simulink model "pasp_reordertest"  (Simulink 6.2)
settings: Solver=ode45  StartTime=0.0  StopTime=30000  RelTol=1e-3
undefined symbols (not defined in the file or in its folder): iBOB
libraries: xbsIndex_r3 x1464, casper_library x144, xps_library x60
(part 2 of 13)

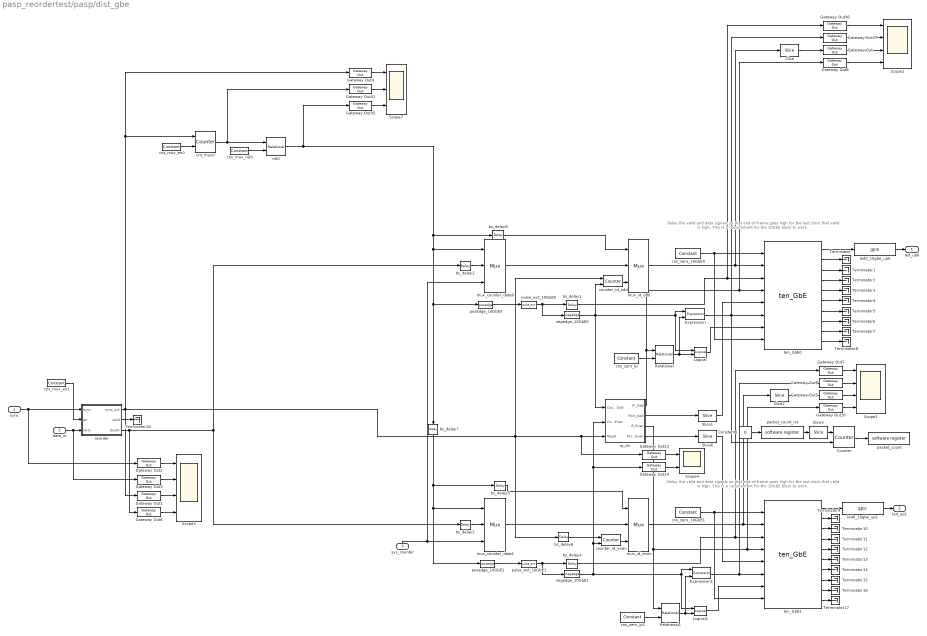
== system pasp_reordertest/pasp/dist_gbe ==
  note: Delay the valid and data signals so that
      | end-of-frame goes high for the last clock
      | that valid is high. This is a requirement for
      | the 10GbE block to work.
  note: Delay the valid and data signals so that
      | end-of-frame goes high for the last clock
      | that valid is high. This is a requirement for
      | the 10GbE block to work.
  sync : Inport  Port=1  LatchInput=off
  data_in : Inport  Port=2  LatchInput=off
  sys_counter : Inport  Orientation=up  Port=3  LatchInput=off
  Constant6 : Constant  Value=0
  Counter : xbsIndex_r3/Counter  cnt_type=Free Running  n_bits=32  bin_pt=0  arith_type=Unsigned  start_count=0  cnt_to=Inf  cnt_by_val=1  operation=Up  explicit_period=off  period=1  load_pin=off  rst=on  en=on  dbl_ovrd=off  show_param=off  use_rpm=on  gen_core=off
      settings: xl_area=[0, 0, 0, 0, 0, 0, 0]
  Expression : xbsIndex_r3/Expression  expression=a & ~b  precision=Full  arith_type=Unsigned  n_bits=8  bin_pt=2  align_bp=on  latency=0  explicit_period=off  period=1  en=off  dbl_ovrd=off  show_param=off
      settings: xl_area=[0, 0, 0, 0, 0, 0, 0]
  Expression1 : xbsIndex_r3/Expression  expression=a & ~b  precision=Full  arith_type=Unsigned  n_bits=8  bin_pt=2  align_bp=on  latency=0  explicit_period=off  period=1  en=off  dbl_ovrd=off  show_param=off
      settings: xl_area=[0, 0, 0, 0, 0, 0, 0]
  Gateway Out{,1..10,13..14,31,35..37} (17 alike) : xbsIndex_r3/Gateway Out  output_type=Double  nbits=8  bin_pt=6  arith_type=Boolean  quantization=Truncate  overflow=Wrap  hdl_port=on  timing_constraint=None  locs_specified=off  LOCs={}  needs_fixed_name=off  show_param=off
      settings: xl_area=[0, 0, 0, 0, 0, 0, 0]
  Logical : xbsIndex_r3/Logical  logical_function=AND  inputs=2  precision=Full  arith_type=Unsigned  n_bits=8  bin_pt=2  align_bp=on  latency=0  explicit_period=off  period=1  en=off  dbl_ovrd=off  show_param=off
      settings: xl_area=[0, 0, 0, 0, 0, 0, 0]
  Logical1 : xbsIndex_r3/Logical  logical_function=AND  inputs=2  precision=Full  arith_type=Unsigned  n_bits=8  bin_pt=2  align_bp=on  latency=0  explicit_period=off  period=1  en=off  dbl_ovrd=off  show_param=off
      settings: xl_area=[0, 0, 0, 0, 0, 0, 0]
  Relational : xbsIndex_r3/Relational  mode=a=b  latency=1  explicit_period=off  period=1  en=off  dbl_ovrd=off  show_param=off
      settings: xl_area=[0, 0, 0, 0, 0, 0, 0]
  Relational1 : xbsIndex_r3/Relational  mode=a=b  latency=1  explicit_period=off  period=1  en=off  dbl_ovrd=off  show_param=off
      settings: xl_area=[0, 0, 0, 0, 0, 0, 0]
  Scope1 : Scope  NumInputPorts=4
      settings: TimeRange=10000  YMin=0~0~0~4000  YMax=1~1~16~4016
  Scope2 : Scope  NumInputPorts=4
      settings: TimeRange=10000  YMin=0~0~0~0  YMax=1~1~10000~6.5e+010  SaveName=ScopeData2
  Scope3 : Scope  NumInputPorts=4
      settings: TimeRange=6000  YMin=0~0~-1~0  YMax=1~65~1~65  SaveName=ScopeData4
  Scope4 : Scope  NumInputPorts=2
      settings: TimeRange=10000  YMin=0~0  YMax=1~1  SaveName=ScopeData6
  Scope7 : Scope  NumInputPorts=3
      settings: YMin=0~0~0  YMax=1~275~1
  Slice : xbsIndex_r3/Slice  mode=Lower Bit Location + Width  nbits=5  bit1=0  base1=MSB of Input  bit0=0  base0=LSB of Input  boolean_output=off  explicit_period=off  period=1  dbl_ovrd=off
  Slice1 : xbsIndex_r3/Slice  mode=Lower Bit Location + Width  nbits=16  bit1=0  base1=MSB of Input  bit0=0  base0=LSB of Input  boolean_output=off  explicit_period=off  period=1  dbl_ovrd=off
  Slice2 : xbsIndex_r3/Slice  mode=Lower Bit Location + Width  nbits=5  bit1=0  base1=MSB of Input  bit0=0  base0=LSB of Input  boolean_output=off  explicit_period=off  period=1  dbl_ovrd=off
  Slice3 : xbsIndex_r3/Slice  mode=Lower Bit Location + Width  nbits=1  bit1=0  base1=MSB of Input  bit0=0  base0=LSB of Input  boolean_output=on  explicit_period=off  period=1  dbl_ovrd=off
  Slice6 : xbsIndex_r3/Slice  mode=Lower Bit Location + Width  nbits=16  bit1=0  base1=MSB of Input  bit0=0  base0=LSB of Input  boolean_output=off  explicit_period=off  period=1  dbl_ovrd=off
  Terminator{,1..18} (19 alike) : Terminator
  bs_delay{1..2,4..5} (4 alike) : xbsIndex_r3/Delay  latency=1  reg_retiming=off  explicit_period=on  period=1  en=off  accept_only_valid=off  init_zero=on  dbl_ovrd=off  show_param=off
      settings: xl_area=[0, 0, 0, 0, 0, 0, 0]
  bs_delay3 : xbsIndex_r3/Delay  latency=2  reg_retiming=off  explicit_period=on  period=1  en=off  accept_only_valid=off  init_zero=on  dbl_ovrd=off  show_param=off
      settings: xl_area=[0, 0, 0, 0, 0, 0, 0]
  bs_delay6 : xbsIndex_r3/Delay  latency=4  reg_retiming=off  explicit_period=on  period=1  en=off  accept_only_valid=off  init_zero=on  dbl_ovrd=off  show_param=off
      settings: xl_area=[0, 0, 0, 0, 0, 0, 0]
  bs_delay7 : xbsIndex_r3/Delay  Orientation=down  latency=256  reg_retiming=off  explicit_period=on  period=1  en=off  accept_only_valid=off  init_zero=on  dbl_ovrd=off  show_param=off
      settings: xl_area=[0, 0, 0, 0, 0, 0, 0]
  bs_delay8 : xbsIndex_r3/Delay  latency=2  reg_retiming=off  explicit_period=on  period=1  en=off  accept_only_valid=off  init_zero=on  dbl_ovrd=off  show_param=off
      settings: xl_area=[0, 0, 0, 0, 0, 0, 0]
  cns_mux_en0 : xbsIndex_r3/Constant  const=1  equ=P=C  arith_type=Boolean  n_bits=1  bin_pt=0  opselect=C  inp2=PCIN>>17  opr=+  inp1=P  carry=CIN  iostate=0  explicit_period=on  period=1  dbl_ovrd=off
  cns_mux_en1 : xbsIndex_r3/Constant  const=1  equ=P=C  arith_type=Boolean  n_bits=1  bin_pt=0  opselect=C  inp2=PCIN>>17  opr=+  inp1=P  carry=CIN  iostate=0  explicit_period=on  period=1  dbl_ovrd=off
  cns_mux_rel0 : xbsIndex_r3/Constant  const=510  equ=P=C  arith_type=Unsigned  n_bits=9  bin_pt=0  opselect=C  inp2=PCIN>>17  opr=+  inp1=P  carry=CIN  iostate=0  explicit_period=on  period=1  dbl_ovrd=off
  cns_zero_10GbE0 : xbsIndex_r3/Constant  const=0  equ=P=C  arith_type=Boolean  n_bits=32  bin_pt=0  opselect=C  inp2=PCIN>>17  opr=+  inp1=P  carry=CIN  iostate=0  explicit_period=on  period=1  dbl_ovrd=off
  cns_zero_10GbE1 : xbsIndex_r3/Constant  const=0  equ=P=C  arith_type=Boolean  n_bits=32  bin_pt=0  opselect=C  inp2=PCIN>>17  opr=+  inp1=P  carry=CIN  iostate=0  explicit_period=on  period=1  dbl_ovrd=off
  cns_zero_ip : xbsIndex_r3/Constant  const=0  equ=P=C  arith_type=Unsigned  n_bits=32  bin_pt=0  opselect=C  inp2=PCIN>>17  opr=+  inp1=P  carry=CIN  iostate=0  explicit_period=on  period=1  dbl_ovrd=off
  cns_zero_ip1 : xbsIndex_r3/Constant  const=0  equ=P=C  arith_type=Unsigned  n_bits=32  bin_pt=0  opselect=C  inp2=PCIN>>17  opr=+  inp1=P  carry=CIN  iostate=0  explicit_period=on  period=1  dbl_ovrd=off
  cnt_mux0 : xbsIndex_r3/Counter  cnt_type=Free Running  n_bits=9  bin_pt=0  arith_type=Unsigned  start_count=0  cnt_to=Inf  cnt_by_val=1  operation=Up  explicit_period=off  period=1  load_pin=off  rst=on  en=on  dbl_ovrd=off  show_param=off  use_rpm=on  gen_core=off
      settings: xl_area=[0, 0, 0, 0, 0, 0, 0]
  counter_id_even : xbsIndex_r3/Counter  cnt_type=Count Limited  n_bits=64  bin_pt=0  arith_type=Unsigned  start_count=2  cnt_to=16  cnt_by_val=2  operation=Up  explicit_period=off  period=1  load_pin=off  rst=on  en=on  dbl_ovrd=off  show_param=off  use_rpm=on  gen_core=off
      settings: xl_area=[0, 0, 0, 0, 0, 0, 0]
  counter_id_odd : xbsIndex_r3/Counter  cnt_type=Count Limited  n_bits=64  bin_pt=0  arith_type=Unsigned  start_count=1  cnt_to=15  cnt_by_val=2  operation=Up  explicit_period=off  period=1  load_pin=off  rst=on  en=on  dbl_ovrd=off  show_param=off  use_rpm=on  gen_core=off
      settings: xl_area=[0, 0, 0, 0, 0, 0, 0]
  ip_ctr : Subsystem  mask(ip_ctr){numcomputers=16}
      mask prompts: numcomputers "Num IPs (Must be power of 2)"
      mask init:
      | ip_ctr_init(gcb,...
      |     'numcomputers',numcomputers)
      settings: AttributesFormatString=IPs=16
  led0_10gbe_up0 : xps_library/gpio  Tag=xps:gpio  io_group=iBOB:led  io_dir=out  arith_type=Boolean  bitwidth=1  bin_pt=0  bit_index=1  sample_period=1  use_single_ended=off  use_ddr=off  reg_iob=on  reg_clk_phase=0  termination=None
  led0_10gbe_up1 : xps_library/gpio  Tag=xps:gpio  io_group=iBOB:led  io_dir=out  arith_type=Boolean  bitwidth=1  bin_pt=0  bit_index=2  sample_period=1  use_single_ended=off  use_ddr=off  reg_iob=on  reg_clk_phase=0  termination=None
  mux_counter_data0 : xbsIndex_r3/Mux  inputs=2  precision=Full  arith_type="Signed  (2's comp)"  n_bits=8  bin_pt=2  quantization=Truncate  overflow=Wrap  latency=1  explicit_period=off  period=1  en=off  dbl_ovrd=off  show_param=off  mux_type=off  use_rpm=off  gen_core=off
      settings: xl_area=[0, 0, 0, 0, 0, 0, 0]
  mux_counter_data1 : xbsIndex_r3/Mux  inputs=2  precision=Full  arith_type="Signed  (2's comp)"  n_bits=8  bin_pt=2  quantization=Truncate  overflow=Wrap  latency=1  explicit_period=off  period=1  en=off  dbl_ovrd=off  show_param=off  mux_type=off  use_rpm=off  gen_core=off
      settings: xl_area=[0, 0, 0, 0, 0, 0, 0]
  mux_id_even : xbsIndex_r3/Mux  inputs=2  precision=Full  arith_type="Signed  (2's comp)"  n_bits=8  bin_pt=2  quantization=Truncate  overflow=Wrap  latency=1  explicit_period=off  period=1  en=off  dbl_ovrd=off  show_param=off  mux_type=off  use_rpm=off  gen_core=off
      settings: xl_area=[0, 0, 0, 0, 0, 0, 0]
  mux_id_odd : xbsIndex_r3/Mux  inputs=2  precision=Full  arith_type="Signed  (2's comp)"  n_bits=8  bin_pt=2  quantization=Truncate  overflow=Wrap  latency=1  explicit_period=off  period=1  en=off  dbl_ovrd=off  show_param=off  mux_type=off  use_rpm=off  gen_core=off
      settings: xl_area=[0, 0, 0, 0, 0, 0, 0]
  negedge_10GbE0 : casper_library/Misc/negedge  Tag=Rising Edge Detector
  negedge_10GbE1 : casper_library/Misc/negedge  Tag=Rising Edge Detector
  packet_count : xps_library/software register  Tag=xps:sw_reg  io_dir=To Processor  arith_type=Unsigned  bitwidth=32  bin_pt=0  sample_period=1  gw_name=pasp_16i16c128s_pasp_dist_gbe_packet_count_user_data_in
  packet_count_rst : xps_library/software register  Tag=xps:sw_reg  io_dir=From Processor  arith_type=Unsigned  bitwidth=32  bin_pt=0  sample_period=1  gw_name=pasp_16i16c128s_pasp_dist_gbe_packet_count_rst_user_data_out
  posedge_10GbE0 : casper_library/Misc/posedge  Tag=Rising Edge Detector
  posedge_10GbE1 : casper_library/Misc/posedge  Tag=Rising Edge Detector
  pulse_ext_10GbE0 : casper_library/Misc/pulse_ext  pulse_len=258
  pulse_ext_10GbE1 : casper_library/Misc/pulse_ext  pulse_len=258
  rel0 : xbsIndex_r3/Relational  mode=a=b  latency=1  explicit_period=off  period=1  en=off  dbl_ovrd=off  show_param=off
      settings: xl_area=[0, 0, 0, 0, 0, 0, 0]
  reorder : Subsystem  AncestorBlock=casper_library/Reorder/reorder  mask(reorder){map=[0 16 32 48 64 80 96 112 128 144 160 176 192 208 224 240 256 272 288 304 320 336 352 368 384 400 416 432 448 464 480 496 512 528 544 560 576 592 608 624 640 656 672 688 704 720 736 752 768 784 800 816 832 848 864 880 896 912 928 944 960 976 992 1008 1024 1040 1056 1072 1088 1104 1120 1136 1152 1168 1184 1200 1216 1232 1248 1264 1280 1296 1312 1328 1344 1360 1376 1392 1408 1424 1440 1456 1472 1488 1504 1520 1536 1552 1568 1584 1600 1616 1632 1648 1664 1680 1696 1712 1728 1744 1760 1776 1792 1808 1824 1840 1856 1872 1888 1904 1920 1936 1952 1968 1984 2000 2016 2032 2048 2064 2080 2096 2112 2128 2144 2160 2176 2192 2208 2224 2240 2256 2272 2288 2304 2320 2336 2352 2368 2384 2400 2416 2432 2448 2464 2480 2496 2512 2528 2544 2560 2576 2592 2608 2624 2640 2656 2672 2688 2704 2720 2736 2752 2768 2784 2800 2816 2832 2848 2864 2880 2896 2912 2928 2944 2960 2976 2992 3008 3024 3040 3056 3072 3088 3104 3120 3136 3152 3168 3184 3200 3216 3232 3248 3264 3280 3296 3312 3328 3344 3360 3376 3392 3408 3424 3440 3456 3472 3488 3504 3520 3536 3552 3568 3584 3600 3616 3632 3648 3664 3680 3696 3712 3728 3744 3760 3776 3792 3808 3824 3840 3856 3872 3888 3904 3920 3936 3952 3968 3984 4000 4016 4032 4048 4064 4080 1 17 33 49 65 81 97 113 129 145 161 177 193 209 225 241 257 273 289 305 321 337 353 369 385 401 417 433 449 465 481 497 513 529 545 561 577 593 609 625 641 657 673 689 705 721 737 753 769 785 801 817 833 849 865 881 897 913 929 945 961 977 993 1009 1025 1041 1057 1073 1089 1105 1121 1137 1153 1169 1185 1201 1217 1233 1249 1265 1281 1297 1313 1329 1345 1361 1377 1393 1409 1425 1441 1457 1473 1489 1505 1521 1537 1553 1569 1585 1601 1617 1633 1649 1665 1681 1697 1713 1729 1745 1761 1777 1793 1809 1825 1841 1857 1873 1889 1905 1921 1937 1953 1969 1985 2001 2017 2033 2049 2065 2081 2097 2113 2129 2145 2161 2177 2193 2209 2225 2241 2257 2273 2289 2305 2321 2337 2353 2369 2385 2401 2417 2433 2449 2465 2481 2497 2513 2529 2545 2561 2577 2593 2609 2625 2641 2657 2673 2689 2705 2721 2737 2753 2769 2785 2801 2817 2833 2849 2865 2881 2897 2913 2929 2945 2961 2977 2993 3009 3025 3041 3057 3073 3089 3105 3121 3137 3153 3169 3185 3201 3217 3233 3249 3265 3281 3297 3313 3329 3345 3361 3377 3393 3409 3425 3441 3457 3473 3489 3505 3521 3537 3553 3569 3585 3601 3617 3633 3649 3665 3681 3697 3713 3729 3745 3761 3777 3793 3809 3825 3841 3857 3873 3889 3905 3921 3937 3953 3969 3985 4001 4017 4033 4049 4065 4081 2 18 34 50 66 82 98 114 130 146 162 178 194 210 226 242 258 274 290 306 322 338 354 370 386 402 418 434 450 466 482 498 514 530 546 562 578 594 610 626 642 658 674 690 706 722 738 754 770 786 802 818 834 850 866 882 898 914 930 946 962 978 994 1010 1026 1042 1058 1074 1090 1106 1122 1138 1154 1170 1186 1202 1218 1234 1250 1266 1282 1298 1314 1330 1346 1362 1378 1394 1410 1426 1442 1458 1474 1490 1506 1522 1538 1554 1570 1586 1602 1618 1634 1650 1666 1682 1698 1714 1730 1746 1762 1778 1794 1810 1826 1842 1858 1874 1890 1906 1922 1938 1954 1970 1986 2002 2018 2034 2050 2066 2082 2098 2114 2130 2146 2162 2178 2194 2210 2226 2242 2258 2274 2290 2306 2322 2338 2354 2370 2386 2402 2418 2434 2450 2466 2482 2498 2514 2530 2546 2562 2578 2594 2610 2626 2642 2658 2674 2690 2706 2722 2738 2754 2770 2786 2802 2818 2834 2850 2866 2882 2898 2914 2930 2946 2962 2978 2994 3010 3026 3042 3058 3074 3090 3106 3122 3138 3154 3170 3186 3202 3218 3234 3250 3266 3282 3298 3314 3330 3346 3362 3378 3394 3410 3426 3442 3458 3474 3490 3506 3522 3538 3554 3570 3586 3602 3618 3634 3650 3666 3682 3698 3714 3730 3746 3762 3778 3794 3810 3826 3842 3858 3874 3890 3906 3922 3938 3954 3970 3986 4002 4018 4034 4050 4066 4082 3 19 35 51 67 83 99 115 131 147 163 179 195 211 227 243 259 275 291 307 323 339 355 371 387 403 419 435 451 467 483 499 515 531 547 563 579 595 611 627 643 659 675 691 707 723 739 755 771 787 803 819 835 851 867 883 899 915 931 947 963 979 995 1011 1027 1043 1059 1075 1091 1107 1123 1139 1155 1171 1187 1203 1219 1235 1251 1267 1283 1299 1315 1331 1347 1363 1379 1395 ...(+15374 chars)], n_inputs=1, bram_latency=2, map_latency=1, double_buffer=0}
      mask prompts: map "Output Order:"; n_inputs "Number of inputs"; bram_latency "BRAM Latency"; map_latency "Map Latency"; double_buffer "Double Buffer"
      mask init:
      | reorder_init(gcb, ...
      |     'map', map, ...
      |     'n_inputs', n_inputs, ...
      |     'bram_latency', bram_latency, ...
      |     'map_latency', map_latency, ...
      |     'double_buffer', double_buffer);
      settings: AttributesFormatString=order=3
  ten_GbE0 : xps_library/ten_GbE  Tag=xps:tengbe  port=iBOB:0  mac_lite=on  show_param=on  pre_emph=2  swing=800
  ten_GbE1 : xps_library/ten_GbE  Tag=xps:tengbe  port=iBOB:1  mac_lite=on  show_param=on  pre_emph=2  swing=800
  led_up0 : Outport
  led_up1 : Outport  Port=2
  wires:
  sys_counter/1 -> mux_counter_data1/3, mux_counter_data0/3
  data_in/1 -> Gateway Out3/1, reorder/3(din0)
  reorder/2(valid) -> Terminator18/1
  Gateway Out36/1 -> Scope1/1
  ten_GbE1/10 -> Terminator17/1
  ten_GbE1/9 -> Terminator16/1
  ten_GbE1/8 -> Terminator15/1
  ten_GbE1/7 -> Terminator14/1
  ten_GbE1/6 -> Terminator13/1
  ten_GbE1/5 -> Terminator12/1
  ten_GbE1/4 -> Terminator11/1
  ten_GbE1/3 -> Terminator10/1
  ten_GbE1/2 -> Terminator9/1
  ten_GbE0/10 -> Terminator8/1
  ten_GbE0/9 -> Terminator7/1
  ten_GbE0/8 -> Terminator6/1
  ten_GbE0/7 -> Terminator5/1
  ten_GbE0/6 -> Terminator4/1
  ten_GbE0/5 -> Terminator3/1
  ten_GbE0/4 -> Terminator2/1
  ten_GbE0/3 -> Terminator1/1
  ten_GbE0/2 -> Terminator/1
  ten_GbE0/1 -> led0_10gbe_up0/1
  cns_zero_10GbE0/1 -> ten_GbE0/1, ten_GbE0/8
  mux_counter_data0/1 -> mux_id_odd/2
  cnt_mux0/1 -> rel0/1, Gateway Out31/1
  cns_mux_en0/1 -> cnt_mux0/2
  Gateway Out37/1 -> Scope1/2
  Gateway Out/1 -> Scope1/3
  pulse_ext_10GbE0/1 -> bs_delay1/1, negedge_10GbE0/1
  negedge_10GbE0/1 -> Logical/1, Expression/1, ip_ctr/1(Count_Odd), counter_id_odd/2
  cns_mux_rel0/1 -> rel0/2
  rel0/1 -> Gateway Out35/1, mux_counter_data0/1, posedge_10GbE0/1, bs_delay7/1, bs_delay8/1
  posedge_10GbE0/1 -> pulse_ext_10GbE0/1
  bs_delay1/1 -> ten_GbE0/3, Gateway Out36/1
  mux_id_odd/1 -> ten_GbE0/2, Slice/1
  Gateway Out4/1 -> Scope7/1
  Gateway Out31/1 -> Scope7/2
  Gateway Out35/1 -> Scope7/3
  bs_delay2/1 -> mux_counter_data0/2
  ten_GbE1/1 -> led0_10gbe_up1/1
  cns_zero_10GbE1/1 -> ten_GbE1/1, ten_GbE1/8
  mux_counter_data1/1 -> mux_id_even/2
  pulse_ext_10GbE1/1 -> negedge_10GbE1/1, bs_delay4/1
  negedge_10GbE1/1 -> Logical1/1, Expression1/1, counter_id_even/2, ip_ctr/2(Count_Even), Gateway Out14/1
  posedge_10GbE1/1 -> pulse_ext_10GbE1/1
  bs_delay4/1 -> ten_GbE1/3, Gateway Out7/1
  mux_id_even/1 -> ten_GbE1/2, Slice2/1
  bs_delay5/1 -> mux_counter_data1/2
  bs_delay7/1 -> mux_counter_data1/1, posedge_10GbE1/1, bs_delay3/1
  Gateway Out9/1 -> Scope2/2
  reorder/3(dout0) -> bs_delay5/1, bs_delay2/1, Gateway Out6/1
  cns_mux_en1/1 -> reorder/2(en)
  Gateway Out2/1 -> Scope3/1
  Gateway Out3/1 -> Scope3/2
  Gateway Out1/1 -> Scope3/3
  Gateway Out6/1 -> Scope3/4
  reorder/1(sync_out) -> Gateway Out1/1, cnt_mux0/1, Gateway Out4/1, counter_id_odd/1, ip_ctr/3(Reset), Gateway Out13/1, bs_delay6/1
  sync/1 -> reorder/1(sync), Gateway Out2/1
  led0_10gbe_up0/1 -> led_up0/1
  led0_10gbe_up1/1 -> led_up1/1
  cns_zero_ip/1 -> Relational/2
  Logical/1 -> ten_GbE0/7
  Relational/1 -> Logical/2, Expression/2
  Expression/1 -> ten_GbE0/6, Gateway Out37/1, Counter/2
  Relational1/1 -> Logical1/2, Expression1/2
  Logical1/1 -> ten_GbE1/7
  Expression1/1 -> ten_GbE1/6, Gateway Out9/1
  cns_zero_ip1/1 -> Relational1/2
  Gateway Out8/1 -> Scope1/4
  Slice/1 -> Gateway Out/1
  ip_ctr/2(Port_Odd) -> Slice1/1
  Slice1/1 -> ten_GbE0/5
  Slice6/1 -> ten_GbE1/5
  Slice2/1 -> Gateway Out5/1
  ip_ctr/4(Port_Even) -> Slice6/1
  ip_ctr/1(IP_Odd) -> Relational/1, ten_GbE0/4, Gateway Out8/1
  Gateway Out7/1 -> Scope2/1
  Gateway Out5/1 -> Scope2/3
  Gateway Out10/1 -> Scope2/4
  bs_delay8/1 -> mux_id_odd/1
  counter_id_odd/1 -> mux_id_odd/3
  bs_delay3/1 -> mux_id_even/1
  counter_id_even/1 -> mux_id_even/3
  Gateway Out14/1 -> Scope4/2
  Gateway Out13/1 -> Scope4/1
  ip_ctr/3(IP_Even) -> Relational1/1, ten_GbE1/4, Gateway Out10/1
  bs_delay6/1 -> counter_id_even/1
  Counter/1 -> packet_count/1
  packet_count_rst/1 -> Slice3/1
  Slice3/1 -> Counter/1
  Constant6/1 -> packet_count_rst/1

== system pasp_reordertest/pasp/fft_wideband_real ==
  sync : Inport  Port=1  LatchInput=off
  shift : Inport  Port=2  LatchInput=off
  in0 : Inport  Port=3  LatchInput=off
  in1 : Inport  Port=4  LatchInput=off
  in2 : Inport  Port=5  LatchInput=off
  in3 : Inport  Port=6  LatchInput=off
  fft_biplex_real_4x0 : Subsystem  AncestorBlock=casper_library/FFTs/fft_biplex_real_4x  mask(fft_biplex_real_4x){FFTSize=3, BitWidth=18, quantization=Truncate, overflow=Wrap, add_latency=2, mult_latency=3, bram_latency=2}
      mask prompts: FFTSize "Size of FFT: (2^? pnts)"; BitWidth "Bitwidth: (Max Efficiency at 18 bits)"; quantization "Quantization Behavior"; overflow "Overflow Behavior"; add_latency "Add Latency"; mult_latency "Mult Latency"; bram_latency "BRAM Latency"
      mask init:
      | fft_biplex_real_4x_init(gcb,...
      |     'FFTSize', FFTSize,...
      |     'BitWidth', BitWidth,...
      |     'quantization', quantization,...
      |     'overflow', overflow,...
      |     'add_latency', add_latency,...
      |     'mult_latency', mult_latency,...
      |     'bram_latency', bram_latency);
      settings: AttributesFormatString=FFTSize=3, BitWidth=18
      mask StyleString: edit,edit,popup(Truncate|Round  (unbiased: +/- Inf)|Round  (unbiased: Even Values)),popup(Wrap|Saturate|Error),edit,edit,edit
  fft_direct : Subsystem  AncestorBlock=casper_library/FFTs/fft_direct  mask(fft_direct){FFTSize=2, BitWidth=18, add_latency=2, mult_latency=3, bram_latency=2, quantization=Truncate, overflow=Wrap, MapTail=1, LargerFFTSize=5, StartStage=4}
      mask prompts: FFTSize "Size of FFT: (2^?)"; BitWidth "Bit Width"; add_latency "Add Latency"; mult_latency "Mult Latency"; bram_latency "BRAM Latency"; quantization "Quantization Behavior"; overflow "Overflow Behavior"; MapTail "Map Tail of Larger FFT"; LargerFFTSize "Size of Larger FFT (2^?):"; StartStage "Start Stage of Map Tail:"
      mask init:
      | fft_direct_init(gcb,...
      |     'FFTSize', FFTSize,...
      |     'BitWidth', BitWidth,...
      |     'add_latency', add_latency,...
      |     'mult_latency', mult_latency,...
      |     'bram_latency', bram_latency,...
      |     'quantization', quantization,...
      |     'overflow', overflow,...
      |     'MapTail', MapTail,...
      |     'LargerFFTSize', LargerFFTSize,...
      |     'StartStage', StartStage);
      settings: AttributesFormatString=FFTSize=2
      mask StyleString: edit,edit,edit,edit,edit,popup(Truncate|Round  (unbiased: +/- Inf)|Round  (unbiased: Even Values)),popup(Wrap|Saturate|Error),edit,edit,edit
  fft_unscrambler : Subsystem  AncestorBlock=casper_library/FFTs/fft_unscrambler  mask(fft_unscrambler){FFTSize=4, n_inputs=1, bram_latency=2}
      mask prompts: FFTSize "Size of FFT: (2^?)"; n_inputs "Number of Simultaneous Inputs: (2^?)"; bram_latency "BRAM Latency"
      mask init:
      | fft_unscrambler_init(gcb,...
      |     'FFTSize',FFTSize,... 
      |     'n_inputs', n_inputs,...
      |     'bram_latency', bram_latency);
      settings: AttributesFormatString=FFTSize=4, n_inputs=1
  slice : xbsIndex_r3/Slice  mode=Lower Bit Location + Width  nbits=2  bit1=0  base1=MSB of Input  bit0=3  base0=LSB of Input  boolean_output=off  explicit_period=off  period=1  dbl_ovrd=off
  sync_out : Outport
  out0 : Outport  Port=2
  out1 : Outport  Port=3
  wires:
  in0/1 -> fft_biplex_real_4x0/1(pol1)
  in1/1 -> fft_biplex_real_4x0/2(pol2)
  in2/1 -> fft_biplex_real_4x0/3(pol3)
  in3/1 -> fft_biplex_real_4x0/4(pol4)
  shift/1 -> fft_biplex_real_4x0/6(shift), slice/1
  sync/1 -> fft_biplex_real_4x0/5(sync)
  slice/1 -> fft_direct/2(shift)
  fft_biplex_real_4x0/6(sync_out) -> fft_direct/1(sync)
  fft_biplex_real_4x0/1(pol1_out) -> fft_direct/3(in0)
  fft_biplex_real_4x0/2(pol2_out) -> fft_direct/4(in1)
  fft_biplex_real_4x0/3(pol3_out) -> fft_direct/5(in2)
  fft_biplex_real_4x0/4(pol4_out) -> fft_direct/6(in3)
  fft_direct/1(sync_out) -> fft_unscrambler/1(sync)
  fft_unscrambler/1(sync_out) -> sync_out/1
  fft_direct/2(out0) -> fft_unscrambler/2(In1)
  fft_unscrambler/2(Out1) -> out0/1
  fft_direct/3(out1) -> fft_unscrambler/3(In2)
  fft_unscrambler/3(Out2) -> out1/1

== system pasp_reordertest/pasp/fft_wideband_real1 ==
  sync : Inport  Port=1  LatchInput=off
  shift : Inport  Port=2  LatchInput=off
  in0 : Inport  Port=3  LatchInput=off
  in1 : Inport  Port=4  LatchInput=off
  in2 : Inport  Port=5  LatchInput=off
  in3 : Inport  Port=6  LatchInput=off
  fft_biplex_real_4x0 : Subsystem  AncestorBlock=casper_library/FFTs/fft_biplex_real_4x  mask(fft_biplex_real_4x){FFTSize=3, BitWidth=18, quantization=Truncate, overflow=Wrap, add_latency=2, mult_latency=3, bram_latency=2}
      mask prompts: FFTSize "Size of FFT: (2^? pnts)"; BitWidth "Bitwidth: (Max Efficiency at 18 bits)"; quantization "Quantization Behavior"; overflow "Overflow Behavior"; add_latency "Add Latency"; mult_latency "Mult Latency"; bram_latency "BRAM Latency"
      mask init: same as pasp_reordertest/pasp/fft_wideband_real/fft_biplex_real_4x0
      settings: AttributesFormatString=FFTSize=3, BitWidth=18
      mask StyleString: edit,edit,popup(Truncate|Round  (unbiased: +/- Inf)|Round  (unbiased: Even Values)),popup(Wrap|Saturate|Error),edit,edit,edit
  fft_direct : Subsystem  AncestorBlock=casper_library/FFTs/fft_direct  mask(fft_direct){FFTSize=2, BitWidth=18, add_latency=2, mult_latency=3, bram_latency=2, quantization=Truncate, overflow=Wrap, MapTail=1, LargerFFTSize=5, StartStage=4}
      mask prompts: FFTSize "Size of FFT: (2^?)"; BitWidth "Bit Width"; add_latency "Add Latency"; mult_latency "Mult Latency"; bram_latency "BRAM Latency"; quantization "Quantization Behavior"; overflow "Overflow Behavior"; MapTail "Map Tail of Larger FFT"; LargerFFTSize "Size of Larger FFT (2^?):"; StartStage "Start Stage of Map Tail:"
      mask init: same as pasp_reordertest/pasp/fft_wideband_real/fft_direct
      settings: AttributesFormatString=FFTSize=2
      mask StyleString: edit,edit,edit,edit,edit,popup(Truncate|Round  (unbiased: +/- Inf)|Round  (unbiased: Even Values)),popup(Wrap|Saturate|Error),edit,edit,edit
  fft_unscrambler : Subsystem  AncestorBlock=casper_library/FFTs/fft_unscrambler  mask(fft_unscrambler){FFTSize=4, n_inputs=1, bram_latency=2}
      mask prompts: FFTSize "Size of FFT: (2^?)"; n_inputs "Number of Simultaneous Inputs: (2^?)"; bram_latency "BRAM Latency"
      mask init:
      | fft_unscrambler_init(gcb,...
      |     'FFTSize',FFTSize,... 
      |     'n_inputs', n_inputs,...
      |     'bram_latency', bram_latency);
      settings: AttributesFormatString=FFTSize=4, n_inputs=1
  slice : xbsIndex_r3/Slice  mode=Lower Bit Location + Width  nbits=2  bit1=0  base1=MSB of Input  bit0=3  base0=LSB of Input  boolean_output=off  explicit_period=off  period=1  dbl_ovrd=off
  sync_out : Outport
  out0 : Outport  Port=2
  out1 : Outport  Port=3
  wires:
  in0/1 -> fft_biplex_real_4x0/1(pol1)
  in1/1 -> fft_biplex_real_4x0/2(pol2)
  in2/1 -> fft_biplex_real_4x0/3(pol3)
  in3/1 -> fft_biplex_real_4x0/4(pol4)
  shift/1 -> fft_biplex_real_4x0/6(shift), slice/1
  sync/1 -> fft_biplex_real_4x0/5(sync)
  slice/1 -> fft_direct/2(shift)
  fft_biplex_real_4x0/6(sync_out) -> fft_direct/1(sync)
  fft_biplex_real_4x0/1(pol1_out) -> fft_direct/3(in0)
  fft_biplex_real_4x0/2(pol2_out) -> fft_direct/4(in1)
  fft_biplex_real_4x0/3(pol3_out) -> fft_direct/5(in2)
  fft_biplex_real_4x0/4(pol4_out) -> fft_direct/6(in3)
  fft_direct/1(sync_out) -> fft_unscrambler/1(sync)
  fft_unscrambler/1(sync_out) -> sync_out/1
  fft_direct/2(out0) -> fft_unscrambler/2(In1)
  fft_unscrambler/2(Out1) -> out0/1
  fft_direct/3(out1) -> fft_unscrambler/3(In2)
  fft_unscrambler/3(Out2) -> out1/1
